simulink model "Auto_microgrid_forecasting"  (R2020a)
settings: Solver=VariableStepAuto  StartTime=0.0  StopTime=40  MaxStep=1e-4  RelTol=1e-3
PreLoadFcn:
  | %load('GC_maxRPP_WS12_GHI790_BL330_nomSOC.mat')
InitFcn:
  | run('FC_microgrid_param.m')
  | tic
  | run('CARTinitFcn.m')
StopFcn:
  | toc
undefined symbols (not defined in the file or in its folder): breakpoints1, breakpoints2, cc_kp, cp_table_data, ctrl, D1, Delta, DiscIntNeverNeededParam, DT, FC_BESS, FC_PV_FirstSolar, find_system, Fnom, forecast, GC_mode, gcbh, GHI_rated, libFC_BESS, libFC_PV, LowerLimit, magnitude, oversize, pll_ki, pll_kp, Pmax_PV, Pmax_WT, sps_rtmsupport, timer, Ts, Ts_APC, Ts_Control, Ts_Power, U_rated, UpperLimit
libraries: powerlib x146, simulink x124, powerlib_extras x120, powerlib_meascontrol x94, eePowerMeasurement x28, pi_ctrl x20, simulink_extras x12, eeGeneralControl x10, sps_avr x7, libFSArray x2, libLgBattery x1, spsDieselMotorModel x1
(part 14 of 16)

== system Auto_microgrid_forecasting/FC_PV_FirstSolar/AllStringInverters/PV_Control/InvControl1/CB_Meas2/Filter1 ==
  In1 : Inport
  Discrete 2nd-Order Filter : powerlib_extras/Discrete  Control Blocks/Discrete  2nd-Order Filter  FilterType=Lowpass  Fo=10  Zeta=0.707  Ts=Ts  Initialize=off  Vac_Init=[0.8 -25 60]  Vdc_Init=-0.4  PlotResponse=off  param1=[1 500 1]
      settings: SourceProductBaseCode=PS
  Discrete 2nd-Order Filter1 : powerlib_extras/Discrete  Control Blocks/Discrete  2nd-Order Filter  FilterType=Lowpass  Fo=10  Zeta=0.707  Ts=Ts  Initialize=off  Vac_Init=[0.8 -25 60]  Vdc_Init=-0.4  PlotResponse=off  param1=[1 500 1]
      settings: SourceProductBaseCode=PS
  Mux : Mux  Inputs=2
  Selector1 : Selector  InputPortWidth=3  IndexOptions=Index vector (dialog)  Indices=1  OutputSizes=1
  Selector2 : Selector  InputPortWidth=3  IndexOptions=Index vector (dialog)  Indices=2  OutputSizes=1
  Out1 : Outport  VectorParamsAs1DForOutWhenUnconnected=off
  wires:
  Mux/1 -> Out1/1  "idq0_line_flt"
  Discrete 2nd-Order Filter1/1 -> Mux/2
  Discrete 2nd-Order Filter/1 -> Mux/1
  Selector1/1 -> Discrete 2nd-Order Filter/1
  Selector2/1 -> Discrete 2nd-Order Filter1/1
  In1/1 -> Selector1/1, Selector2/1

== system Auto_microgrid_forecasting/FC_PV_FirstSolar/AllStringInverters/PV_Control/InvControl1/CB_Meas2/PQ_Calculator ==
  note: Copyright (c) 2016 Massachusetts Institute of Technology
      | Permission is hereby granted, free of charge, to any person obtaining a copy of this software and associated documentation files (the "Software"), to deal
      | in the Software without restriction, including without limitation the rights to use, copy, modify, merge, publish, distribute, sublicense, and/or sell copies of the
      | Software, and to permit persons to whom the Software is furnished to do so, subject to the following conditions:
      |
      | THE SOFTWARE IS PROVIDED "AS IS", WITHOUT WARRANTY OF ANY KIND, EXPRESS OR IMPLIED, INCLUDING BUT NOT LIMITED TO THE
      | WARRANTIES OF MERCHANTABILITY, FITNESS FOR A PARTICULAR PURPOSE AND NONINFRINGEMENT. IN NO EVENT SHALL THE AUTHORS
      | OR COPYRIGHT HOLDERS BE LIABLE FOR ANY CLAIM, DAMAGES OR OTHER LIABILITY, WHETHER IN AN ACTION OF CONTRACT, TORT OR
      | OTHERWISE, ARISING FROM, OUT OF OR IN CONNECTION WITH THE SOFTWARE OR THE USE OR OTHER DEALINGS IN THE SOFTWARE
  Vabc : Inport
  Iabc : Inport  Port=2
  3-phase Instantaneous Active & Reactive Power : powerlib_extras/Measurements/3-phase  Instantaneous  Active & Reactive Power
      settings: SourceProductBaseCode=PS
  Demux : Demux  Outputs=2
  Discrete Mean value2 : powerlib_extras/Discrete Measurements/Discrete  Mean value  Freq=60  Vinit=0  Ts=Ts
      settings: SourceProductBaseCode=PS
  Gain10 : Gain  Gain=2/3
  Scope : Scope  NumInputPorts=4
  P - kW : Outport  VectorParamsAs1DForOutWhenUnconnected=off
  Q - kVAR : Outport  Port=2  VectorParamsAs1DForOutWhenUnconnected=off
  wires:
  Gain10/1 -> Scope/4, Demux/1
  3-phase Instantaneous Active & Reactive Power/1 -> Scope/3, Discrete Mean value2/1
  Discrete Mean value2/1 -> Gain10/1
  Vabc/1 -> Scope/1, 3-phase Instantaneous Active & Reactive Power/1
  Iabc/1 -> Scope/2, 3-phase Instantaneous Active & Reactive Power/2
  Demux/1 -> P - kW/1  "kw"
  Demux/2 -> Q - kVAR/1  "kvar"

== system Auto_microgrid_forecasting/FC_PV_FirstSolar/AllStringInverters/PV_Control/InvControl1/Droop/Droop ==
  dfvpq : Inport
  droop : Inport  Port=2
  Constant4 : Constant  Value=2
  Dead Zone : DeadZone  LowerValue=-1.1  UpperValue=1.1  SaturateOnIntegerOverflow=on
  Demux : Demux
  Demux1 : Demux
  Discrete 1st-Order Filter : powerlib_extras/Discrete  Control Blocks/Discrete 1st-Order Filter  FilterType=Lowpass  Tc=1e-3  Ts=Ts  Initialize=off  Vac_Init=[0.8 -25 60]  Vdc_Init=-0.4  PlotResponse=off  param1=[1 500 0.1]
      settings: SourceProductBaseCode=PS
  Discrete 1st-Order Filter1 : powerlib_extras/Discrete  Control Blocks/Discrete 1st-Order Filter  FilterType=Lowpass  Tc=1e-3  Ts=Ts  Initialize=off  Vac_Init=[0.8 -25 60]  Vdc_Init=-0.4  PlotResponse=off  param1=[1 500 0.1]
      settings: SourceProductBaseCode=PS
  Discrete 2nd-Order Filter : powerlib_extras/Discrete  Control Blocks/Discrete  2nd-Order Filter  FilterType=Lowpass  Fo=100  Zeta=0.707  Ts=Ts  Initialize=off  Vac_Init=[0.8 -25 60]  Vdc_Init=-0.4  PlotResponse=off  param1=[1 500 1]
      settings: SourceProductBaseCode=PS
  Discrete 2nd-Order Filter1 : powerlib_extras/Discrete  Control Blocks/Discrete  2nd-Order Filter  FilterType=Lowpass  Fo=100  Zeta=0.707  Ts=Ts  Initialize=off  Vac_Init=[0.8 -25 60]  Vdc_Init=-0.4  PlotResponse=off  param1=[1 500 1]
      settings: SourceProductBaseCode=PS
  Mux1 : Mux
  Product{,1..4} (5 alike) : Product
  Selector : Selector  InputPortWidth=4  IndexOptions=Index vector (dialog)  Indices=[3 4 1 2]  OutputSizes=1
  Sum : Sum  Inputs=|++
  dFvpq_out : Outport  VectorParamsAs1DForOutWhenUnconnected=off
  wires:
  Product4/1 -> Sum/2
  Sum/1 -> Mux1/4
  Constant4/1 -> Product4/2
  Dead Zone/1 -> Product4/1
  Discrete 2nd-Order Filter/1 -> Product/1
  Discrete 2nd-Order Filter1/1 -> Dead Zone/1, Product2/1
  Demux/3 -> Discrete 2nd-Order Filter/1  "p"
  Discrete 1st-Order Filter/1 -> Product1/1
  Demux/2 -> Discrete 1st-Order Filter1/1  "v"
  Demux/1 -> Discrete 1st-Order Filter/1  "f"
  dfvpq/1 -> Demux/1
  Selector/1 -> dFvpq_out/1
  Discrete 1st-Order Filter1/1 -> Product3/1
  Demux/4 -> Discrete 2nd-Order Filter1/1  "q"
  Product1/1 -> Mux1/1  "p"
  Product3/1 -> Mux1/2  "q"
  Product/1 -> Mux1/3  "F"
  Product2/1 -> Sum/1  "v"
  Mux1/1 -> Selector/1
  Demux1/1 -> Product1/2
  Demux1/4 -> Product2/2
  Demux1/3 -> Product/2
  Demux1/2 -> Product3/2
  droop/1 -> Demux1/1

== system Auto_microgrid_forecasting/FC_PV_FirstSolar/AllStringInverters/PV_Control/InvControl1/Droop/ExtractCoefs ==
  In1 : Inport
  Bus Selector8 : BusSelector  OutputSignals=FP_droop,VQ_droop,FP_droop,VQ_droop
  Mux : Mux
  Out1 : Outport  VectorParamsAs1DForOutWhenUnconnected=off
  wires:
  Bus Selector8/1 -> Mux/1  "<FP_droop>"
  Bus Selector8/4 -> Mux/4  "<VQ_droop>"
  Bus Selector8/2 -> Mux/2  "<VQ_droop>"
  Bus Selector8/3 -> Mux/3  "<FP_droop>"
  Mux/1 -> Out1/1
  In1/1 -> Bus Selector8/1

== system Auto_microgrid_forecasting/FC_PV_FirstSolar/AllStringInverters/PV_Control/InvControl1/PLL/DebounceAlternative ==
  In : Inport
  Rst : Inport  Port=2
  Bias : Bias  Bias=-0.5
  Constant1 : Constant  Value=2/Tdb_on
  Constant2 : Constant  Value=2/Tdb_off
  Data Type Conversion : DataTypeConversion
  Delay : Delay  DelayLength=1  InitialCondition=0
  Discrete-Time Integrator : DiscreteIntegrator  IntegratorMethod=Accumulation: Forward Euler  gainval=Tdb_sample  ExternalReset=level  InitialConditionSource=external  InitialCondition=-0.001  SampleTime=Tdb_sample  OutDataTypeStr=double  LimitOutput=on  UpperSaturationLimit=1.001  LowerSaturationLimit=-0.001  ICPrevOutput=DiscIntNeverNeededParam  ICPrevScaledInput=DiscIntNeverNeededParam
  Logical Operator : Logic  Operator=NXOR  AllPortsSameDT=off  OutDataTypeStr=boolean
  Logical Operator1 : Logic  Operator=OR  AllPortsSameDT=off  OutDataTypeStr=boolean
  Logical Operator2 : Logic  Operator=NOT  AllPortsSameDT=off  OutDataTypeStr=boolean
  Logical Operator3 : Logic  AllPortsSameDT=off  OutDataTypeStr=boolean
  Product : Product
  Relay : Relay  OnSwitchValue=1  OffSwitchValue=0
  Switch : Switch  Threshold=0.5
  Out : Outport  VectorParamsAs1DForOutWhenUnconnected=off
  IntOut : Outport  Port=2  VectorParamsAs1DForOutWhenUnconnected=off
  wires:
  Product/1 -> Discrete-Time Integrator/1
  Relay/1 -> Out/1, Delay/1
  Discrete-Time Integrator/1 -> Relay/1, IntOut/1
  Bias/1 -> Product/1
  Constant1/1 -> Switch/1
  Constant2/1 -> Switch/3
  Delay/1 -> Switch/2, Logical Operator3/2, Logical Operator/2
  Logical Operator/1 -> Logical Operator1/1
  Switch/1 -> Product/2
  In/1 -> Logical Operator/1, Bias/1
  Logical Operator1/1 -> Discrete-Time Integrator/2
  Rst/1 -> Logical Operator2/1, Logical Operator1/2
  Logical Operator3/1 -> Data Type Conversion/1
  Logical Operator2/1 -> Logical Operator3/1
  Data Type Conversion/1 -> Discrete-Time Integrator/3

== system Auto_microgrid_forecasting/FC_PV_FirstSolar/AllStringInverters/PV_Control/InvControl1/PLL/PLL (3ph)1 ==
  abc : Inport  PortDimensions=3
  Discrete : Subsystem  DialogController=POWERSYS.PowerSysDialog  mask(Discrete PID Controller){Kp=ParK(1), Ki=ParK(2), Kd=ParK(3), TcD=TcD, Par_Limits=[Flim(2) Flim(1)]*2*pi, Init=2*pi*Par_Init(2), Ts=Ts}
      mask prompts: Kp "Proportional gain (Kp):"; Ki "Integral gain (Ki):"; Kd "Derivative gain (Kd):"; TcD "Time constant for derivative filter (s):"; Par_Limits "Output limits: [ Upper   Lower ]"; Init "Output initial value:"; Ts "Sample time:"
      mask help: This block implements a discrete PID controller.
      mask Display: disp('PID');
  Discrete 2nd-Order Filter : powerlib_extras/Discrete  Control Blocks/Discrete  2nd-Order Filter  FilterType=Lowpass  Fo=10  Zeta=0.707  Ts=Ts  Initialize=off  Vac_Init=[0.8 -25 60]  Vdc_Init=-0.4  PlotResponse=off  param1=[1 500 1]
      settings: SourceProductBaseCode=PS
  Gain10 : Gain  Gain=1/2/pi  SaturateOnIntegerOverflow=on  OutDataTypeStr=Inherit: Same as input  ParamDataTypeStr=Inherit: Same as input
  Mux3 : Mux  Inputs=2
  Scope : Scope  NumInputPorts=4
  Selector : Selector  InputPortWidth=3  IndexOptions=Index vector (dialog)  Indices=2  OutputSizes=1
  Trigonometric Function2 : Trigonometry
  Trigonometric Function3 : Trigonometry  Operator=cos
  Unit Delay : UnitDelay  SampleTime=Ts  HasFrameUpgradeWarning=on
  VCO : Subsystem
  abc_to_dq0 Transformation : powerlib_extras/Measurements/abc_to_dq0 Transformation
      settings: SourceProductBaseCode=PS
  Freq : Outport  VectorParamsAs1DForOutWhenUnconnected=off
  wt : Outport  Port=2  VectorParamsAs1DForOutWhenUnconnected=off
  dq0 : Outport  Port=3  VectorParamsAs1DForOutWhenUnconnected=off
  wires:
  Trigonometric Function3/1 -> Mux3/2
  Trigonometric Function2/1 -> Mux3/1
  Mux3/1 -> abc_to_dq0 Transformation/2  "ejwt"
  abc_to_dq0 Transformation/1 -> dq0/1, Selector/1
  abc/1 -> Scope/4, abc_to_dq0 Transformation/1
  Discrete 2nd-Order Filter/1 -> Unit Delay/1
  Selector/1 -> Scope/1, Discrete/1(Err)  "Vq"
  Gain10/1 -> Discrete 2nd-Order Filter/1
  Unit Delay/1 -> Freq/1
  Discrete/1(Out) -> Scope/2, VCO/1(w), Gain10/1  "W"
  VCO/1(theta) -> Trigonometric Function2/1, Trigonometric Function3/1, wt/1, Scope/3  "wt"

== system Auto_microgrid_forecasting/FC_PV_FirstSolar/AllStringInverters/PV_Control/InvControl1/PLL/VCO ==
  w : Inport
  rst : Inport  Port=2
  init : Inport  Port=3
  Compare To Constant : simulink/Logic and Bit Operations/Compare To Constant  relop=>=  const=pi  OutDataTypeStr=uint8
  Data Type Conversion : DataTypeConversion
  Gain : Gain  Gain=2*pi  OutDataTypeStr=double
  Gain2 : Gain  Gain=Ts  SaturateOnIntegerOverflow=on  OutDataTypeStr=Inherit: Same as input  ParamDataTypeStr=Inherit: Same as input
  Sum : Sum  Inputs=-++
  Switch : Switch  Threshold=0.5
  Unit Delay1 : UnitDelay  SampleTime=-1  HasFrameUpgradeWarning=on
  theta : Outport  VectorParamsAs1DForOutWhenUnconnected=off
  wires:
  Data Type Conversion/1 -> Gain/1
  init/1 -> Switch/1
  rst/1 -> Switch/2
  Switch/1 -> Unit Delay1/1
  Sum/1 -> Switch/3
  Gain2/1 -> Sum/2
  Unit Delay1/1 -> Compare To Constant/1, theta/1, Sum/3  "wt"
  Compare To Constant/1 -> Data Type Conversion/1
  Gain/1 -> Sum/1
  w/1 -> Gain2/1

== system Auto_microgrid_forecasting/FC_PV_FirstSolar/AllStringInverters/PV_Control/InvControl1/Ref_Limiting/RefLimiting ==
  fvpq_in : Inport
  p_max : Inport  Port=2
  p_min : Inport  Port=3
  Complex to Magnitude-Angle : ComplexToMagnitudeAngle
  Complex to Real-Imag : ComplexToRealImag
  Demux : Demux
  Magnitude-Angle to Complex : MagnitudeAngleToComplex
  Mux2 : Mux
  Real-Imag to Complex : RealImagToComplex
  Saturation : Saturate  UpperLimit=1.1  LowerLimit=0.9
  Saturation Dynamic : simulink/Discontinuities/Saturation Dynamic  OutMin=[]  OutMax=[]  OutDataTypeStr=Inherit: Same as second input  OutDataType=fixdt(1, 16)  OutScaling=2^-10  DoSatur=off
  Saturation1 : Saturate  UpperLimit=1.5  LowerLimit=00
  Saturation2 : Saturate  UpperLimit=1  LowerLimit=0
  fvpq_out : Outport  VectorParamsAs1DForOutWhenUnconnected=off
  wires:
  p_min/1 -> Saturation Dynamic/3
  Saturation1/1 -> Mux2/2
  Magnitude-Angle to Complex/1 -> Complex to Real-Imag/1
  Mux2/1 -> fvpq_out/1  "fvpq"
  Demux/3 -> Saturation Dynamic/2
  Saturation Dynamic/1 -> Real-Imag to Complex/1
  Complex to Magnitude-Angle/1 -> Saturation2/1
  Complex to Real-Imag/2 -> Mux2/4
  Complex to Real-Imag/1 -> Mux2/3
  Real-Imag to Complex/1 -> Complex to Magnitude-Angle/1
  Demux/2 -> Saturation1/1
  Demux/1 -> Saturation/1
  fvpq_in/1 -> Demux/1
  Saturation2/1 -> Magnitude-Angle to Complex/1
  Saturation/1 -> Mux2/1
  p_max/1 -> Saturation Dynamic/1
  Complex to Magnitude-Angle/2 -> Magnitude-Angle to Complex/2
  Demux/4 -> Real-Imag to Complex/2

== system Auto_microgrid_forecasting/FC_PV_FirstSolar/AllStringInverters/PV_Control/InvControl2/40_V_Control/Subsystem ==
  in : Inport
  rst : Inport  Port=2
  init : Inport  Port=3
  rate : Inport  Port=4
  Gain : Gain  Gain=[Ts Ts]
  Gain1 : Gain  Gain=-1
  Saturation Dynamic : simulink/Discontinuities/Saturation Dynamic  OutMin=[]  OutMax=[]  OutDataTypeStr=Inherit: Same as second input  OutDataType=fixdt(1, 16)  OutScaling=2^-10  DoSatur=off
  Sum : Sum  Inputs=|++
  Sum1 : Sum  Inputs=-+|
  Switch : Switch  Criteria=u2 > Threshold
  Unit Delay : UnitDelay  SampleTime=-1  HasFrameUpgradeWarning=on
  out : Outport  VectorParamsAs1DForOutWhenUnconnected=off
  wires:
  Switch/1 -> Unit Delay/1
  Sum/1 -> Switch/3
  Saturation Dynamic/1 -> Sum/1
  in/1 -> Sum1/2
  Sum1/1 -> Saturation Dynamic/2
  rst/1 -> Switch/2
  init/1 -> Switch/1
  Unit Delay/1 -> Sum/2, Sum1/1, out/1
  rate/1 -> Gain/1
  Gain/1 -> Saturation Dynamic/1, Gain1/1
  Gain1/1 -> Saturation Dynamic/3

== system Auto_microgrid_forecasting/FC_PV_FirstSolar/AllStringInverters/PV_Control/InvControl2/50_I_Control/Filter ==
  In1 : Inport
  Discrete 2nd-Order Filter : powerlib_extras/Discrete  Control Blocks/Discrete  2nd-Order Filter  FilterType=Lowpass  Fo=300  Zeta=0.707  Ts=Ts  Initialize=off  Vac_Init=[0.8 -25 60]  Vdc_Init=-0.4  PlotResponse=off  param1=[1 500 1]
      settings: SourceProductBaseCode=PS
  Discrete 2nd-Order Filter1 : powerlib_extras/Discrete  Control Blocks/Discrete  2nd-Order Filter  FilterType=Lowpass  Fo=300  Zeta=0.707  Ts=Ts  Initialize=off  Vac_Init=[0.8 -25 60]  Vdc_Init=-0.4  PlotResponse=off  param1=[1 500 1]
      settings: SourceProductBaseCode=PS
  Mux : Mux  Inputs=2
  Selector1 : Selector  InputPortWidth=2  IndexOptions=Index vector (dialog)  Indices=1  OutputSizes=1
  Selector2 : Selector  InputPortWidth=2  IndexOptions=Index vector (dialog)  Indices=2  OutputSizes=1
  Out1 : Outport  VectorParamsAs1DForOutWhenUnconnected=off
  wires:
  In1/1 -> Selector2/1, Selector1/1
  Selector2/1 -> Discrete 2nd-Order Filter1/1
  Selector1/1 -> Discrete 2nd-Order Filter/1
  Discrete 2nd-Order Filter/1 -> Mux/1
  Discrete 2nd-Order Filter1/1 -> Mux/2
  Mux/1 -> Out1/1  "vdq0_line_flt"

== system Auto_microgrid_forecasting/FC_PV_FirstSolar/AllStringInverters/PV_Control/InvControl2/50_I_Control/Filter1 ==
  In1 : Inport
  Discrete 2nd-Order Filter : powerlib_extras/Discrete  Control Blocks/Discrete  2nd-Order Filter  FilterType=Lowpass  Fo=40  Zeta=1  Ts=Ts  Initialize=off  Vac_Init=[0.8 -25 60]  Vdc_Init=-0.4  PlotResponse=off  param1=[1 500 1]
      settings: SourceProductBaseCode=PS
  Discrete 2nd-Order Filter1 : powerlib_extras/Discrete  Control Blocks/Discrete  2nd-Order Filter  FilterType=Lowpass  Fo=40  Zeta=1  Ts=Ts  Initialize=off  Vac_Init=[0.8 -25 60]  Vdc_Init=-0.4  PlotResponse=off  param1=[1 500 1]
      settings: SourceProductBaseCode=PS
  Mux : Mux  Inputs=2
  Selector1 : Selector  InputPortWidth=2  IndexOptions=Index vector (dialog)  Indices=1  OutputSizes=1
  Selector2 : Selector  InputPortWidth=2  IndexOptions=Index vector (dialog)  Indices=2  OutputSizes=1
  Out1 : Outport  VectorParamsAs1DForOutWhenUnconnected=off
  wires:
  Mux/1 -> Out1/1  "vdq0_line_flt"
  Discrete 2nd-Order Filter1/1 -> Mux/2
  Discrete 2nd-Order Filter/1 -> Mux/1
  Selector1/1 -> Discrete 2nd-Order Filter/1
  Selector2/1 -> Discrete 2nd-Order Filter1/1
  In1/1 -> Selector1/1, Selector2/1

== system Auto_microgrid_forecasting/FC_PV_FirstSolar/AllStringInverters/PV_Control/InvControl2/50_I_Control/Subsystem ==
  in : Inport
  rst : Inport  Port=2
  init : Inport  Port=3
  rate : Inport  Port=4
  Gain : Gain  Gain=[Ts Ts]
  Gain1 : Gain  Gain=-1
  Saturation Dynamic : simulink/Discontinuities/Saturation Dynamic  OutMin=[]  OutMax=[]  OutDataTypeStr=Inherit: Same as second input  OutDataType=fixdt(1, 16)  OutScaling=2^-10  DoSatur=off
  Sum : Sum  Inputs=|++
  Sum1 : Sum  Inputs=-+|
  Switch : Switch  Criteria=u2 > Threshold
  Unit Delay : UnitDelay  SampleTime=-1  HasFrameUpgradeWarning=on
  out : Outport  VectorParamsAs1DForOutWhenUnconnected=off
  wires:
  Switch/1 -> Unit Delay/1
  Sum/1 -> Switch/3
  Saturation Dynamic/1 -> Sum/1
  in/1 -> Sum1/2
  Sum1/1 -> Saturation Dynamic/2
  rst/1 -> Switch/2
  init/1 -> Switch/1
  Unit Delay/1 -> Sum/2, Sum1/1, out/1
  rate/1 -> Gain/1
  Gain/1 -> Saturation Dynamic/1, Gain1/1
  Gain1/1 -> Saturation Dynamic/3

== system Auto_microgrid_forecasting/FC_PV_FirstSolar/AllStringInverters/PV_Control/InvControl2/CB_Meas2/Filter ==
  In1 : Inport
  Discrete 2nd-Order Filter : powerlib_extras/Discrete  Control Blocks/Discrete  2nd-Order Filter  FilterType=Lowpass  Fo=10  Zeta=0.707  Ts=Ts  Initialize=off  Vac_Init=[0.8 -25 60]  Vdc_Init=-0.4  PlotResponse=off  param1=[1 500 1]
      settings: SourceProductBaseCode=PS
  Discrete 2nd-Order Filter1 : powerlib_extras/Discrete  Control Blocks/Discrete  2nd-Order Filter  FilterType=Lowpass  Fo=10  Zeta=0.707  Ts=Ts  Initialize=off  Vac_Init=[0.8 -25 60]  Vdc_Init=-0.4  PlotResponse=off  param1=[1 500 1]
      settings: SourceProductBaseCode=PS
  Mux : Mux  Inputs=2
  Selector1 : Selector  InputPortWidth=3  IndexOptions=Index vector (dialog)  Indices=1  OutputSizes=1
  Selector2 : Selector  InputPortWidth=3  IndexOptions=Index vector (dialog)  Indices=2  OutputSizes=1
  Out1 : Outport  VectorParamsAs1DForOutWhenUnconnected=off
  wires:
  In1/1 -> Selector2/1, Selector1/1
  Selector2/1 -> Discrete 2nd-Order Filter1/1
  Selector1/1 -> Discrete 2nd-Order Filter/1
  Discrete 2nd-Order Filter/1 -> Mux/1
  Discrete 2nd-Order Filter1/1 -> Mux/2
  Mux/1 -> Out1/1  "vdq0_line_flt"

== system Auto_microgrid_forecasting/FC_PV_FirstSolar/AllStringInverters/PV_Control/InvControl2/CB_Meas2/Filter1 ==
  In1 : Inport
  Discrete 2nd-Order Filter : powerlib_extras/Discrete  Control Blocks/Discrete  2nd-Order Filter  FilterType=Lowpass  Fo=10  Zeta=0.707  Ts=Ts  Initialize=off  Vac_Init=[0.8 -25 60]  Vdc_Init=-0.4  PlotResponse=off  param1=[1 500 1]
      settings: SourceProductBaseCode=PS
  Discrete 2nd-Order Filter1 : powerlib_extras/Discrete  Control Blocks/Discrete  2nd-Order Filter  FilterType=Lowpass  Fo=10  Zeta=0.707  Ts=Ts  Initialize=off  Vac_Init=[0.8 -25 60]  Vdc_Init=-0.4  PlotResponse=off  param1=[1 500 1]
      settings: SourceProductBaseCode=PS
  Mux : Mux  Inputs=2
  Selector1 : Selector  InputPortWidth=3  IndexOptions=Index vector (dialog)  Indices=1  OutputSizes=1
  Selector2 : Selector  InputPortWidth=3  IndexOptions=Index vector (dialog)  Indices=2  OutputSizes=1
  Out1 : Outport  VectorParamsAs1DForOutWhenUnconnected=off
  wires:
  In1/1 -> Selector2/1, Selector1/1
  Selector2/1 -> Discrete 2nd-Order Filter1/1
  Selector1/1 -> Discrete 2nd-Order Filter/1
  Discrete 2nd-Order Filter/1 -> Mux/1
  Discrete 2nd-Order Filter1/1 -> Mux/2
  Mux/1 -> Out1/1  "idq0_line_flt"

== system Auto_microgrid_forecasting/FC_PV_FirstSolar/AllStringInverters/PV_Control/InvControl2/CB_Meas2/PQ_Calculator ==
  note: Copyright (c) 2016 Massachusetts Institute of Technology
      | Permission is hereby granted, free of charge, to any person obtaining a copy of this software and associated documentation files (the "Software"), to deal
      | in the Software without restriction, including without limitation the rights to use, copy, modify, merge, publish, distribute, sublicense, and/or sell copies of the
      | Software, and to permit persons to whom the Software is furnished to do so, subject to the following conditions:
      |
      | THE SOFTWARE IS PROVIDED "AS IS", WITHOUT WARRANTY OF ANY KIND, EXPRESS OR IMPLIED, INCLUDING BUT NOT LIMITED TO THE
      | WARRANTIES OF MERCHANTABILITY, FITNESS FOR A PARTICULAR PURPOSE AND NONINFRINGEMENT. IN NO EVENT SHALL THE AUTHORS
      | OR COPYRIGHT HOLDERS BE LIABLE FOR ANY CLAIM, DAMAGES OR OTHER LIABILITY, WHETHER IN AN ACTION OF CONTRACT, TORT OR
      | OTHERWISE, ARISING FROM, OUT OF OR IN CONNECTION WITH THE SOFTWARE OR THE USE OR OTHER DEALINGS IN THE SOFTWARE
  Vabc : Inport
  Iabc : Inport  Port=2
  3-phase Instantaneous Active & Reactive Power : powerlib_extras/Measurements/3-phase  Instantaneous  Active & Reactive Power
      settings: SourceProductBaseCode=PS
  Demux : Demux  Outputs=2
  Discrete Mean value2 : powerlib_extras/Discrete Measurements/Discrete  Mean value  Freq=60  Vinit=0  Ts=Ts
      settings: SourceProductBaseCode=PS
  Gain10 : Gain  Gain=2/3
  Scope : Scope  NumInputPorts=4
  P - kW : Outport  VectorParamsAs1DForOutWhenUnconnected=off
  Q - kVAR : Outport  Port=2  VectorParamsAs1DForOutWhenUnconnected=off
  wires:
  Demux/2 -> Q - kVAR/1  "kvar"
  Demux/1 -> P - kW/1  "kw"
  Iabc/1 -> 3-phase Instantaneous Active & Reactive Power/2, Scope/2
  Vabc/1 -> 3-phase Instantaneous Active & Reactive Power/1, Scope/1
  Discrete Mean value2/1 -> Gain10/1
  3-phase Instantaneous Active & Reactive Power/1 -> Discrete Mean value2/1, Scope/3
  Gain10/1 -> Demux/1, Scope/4

== system Auto_microgrid_forecasting/FC_PV_FirstSolar/AllStringInverters/PV_Control/InvControl2/Droop/Droop ==
  dfvpq : Inport
  droop : Inport  Port=2
  Constant4 : Constant  Value=2
  Dead Zone : DeadZone  LowerValue=-1.1  UpperValue=1.1  SaturateOnIntegerOverflow=on
  Demux : Demux
  Demux1 : Demux
  Discrete 1st-Order Filter : powerlib_extras/Discrete  Control Blocks/Discrete 1st-Order Filter  FilterType=Lowpass  Tc=1e-3  Ts=Ts  Initialize=off  Vac_Init=[0.8 -25 60]  Vdc_Init=-0.4  PlotResponse=off  param1=[1 500 0.1]
      settings: SourceProductBaseCode=PS
  Discrete 1st-Order Filter1 : powerlib_extras/Discrete  Control Blocks/Discrete 1st-Order Filter  FilterType=Lowpass  Tc=1e-3  Ts=Ts  Initialize=off  Vac_Init=[0.8 -25 60]  Vdc_Init=-0.4  PlotResponse=off  param1=[1 500 0.1]
      settings: SourceProductBaseCode=PS
  Discrete 2nd-Order Filter : powerlib_extras/Discrete  Control Blocks/Discrete  2nd-Order Filter  FilterType=Lowpass  Fo=100  Zeta=0.707  Ts=Ts  Initialize=off  Vac_Init=[0.8 -25 60]  Vdc_Init=-0.4  PlotResponse=off  param1=[1 500 1]
      settings: SourceProductBaseCode=PS
  Discrete 2nd-Order Filter1 : powerlib_extras/Discrete  Control Blocks/Discrete  2nd-Order Filter  FilterType=Lowpass  Fo=100  Zeta=0.707  Ts=Ts  Initialize=off  Vac_Init=[0.8 -25 60]  Vdc_Init=-0.4  PlotResponse=off  param1=[1 500 1]
      settings: SourceProductBaseCode=PS
  Mux1 : Mux
  Product{,1..4} (5 alike) : Product
  Selector : Selector  InputPortWidth=4  IndexOptions=Index vector (dialog)  Indices=[3 4 1 2]  OutputSizes=1
  Sum : Sum  Inputs=|++
  dFvpq_out : Outport  VectorParamsAs1DForOutWhenUnconnected=off
  wires:
  droop/1 -> Demux1/1
  Demux1/2 -> Product3/2
  Demux1/3 -> Product/2
  Demux1/4 -> Product2/2
  Demux1/1 -> Product1/2
  Mux1/1 -> Selector/1
  Product2/1 -> Sum/1  "v"
  Product/1 -> Mux1/3  "F"
  Product3/1 -> Mux1/2  "q"
  Product1/1 -> Mux1/1  "p"
  Demux/4 -> Discrete 2nd-Order Filter1/1  "q"
  Discrete 1st-Order Filter1/1 -> Product3/1
  Selector/1 -> dFvpq_out/1
  dfvpq/1 -> Demux/1
  Demux/1 -> Discrete 1st-Order Filter/1  "f"
  Demux/2 -> Discrete 1st-Order Filter1/1  "v"
  Discrete 1st-Order Filter/1 -> Product1/1
  Demux/3 -> Discrete 2nd-Order Filter/1  "p"
  Discrete 2nd-Order Filter1/1 -> Product2/1, Dead Zone/1
  Discrete 2nd-Order Filter/1 -> Product/1
  Dead Zone/1 -> Product4/1
  Constant4/1 -> Product4/2
  Sum/1 -> Mux1/4
  Product4/1 -> Sum/2

== system Auto_microgrid_forecasting/FC_PV_FirstSolar/AllStringInverters/PV_Control/InvControl2/Droop/ExtractCoefs ==
  In1 : Inport
  Bus Selector8 : BusSelector  OutputSignals=FP_droop,VQ_droop,FP_droop,VQ_droop
  Mux : Mux
  Out1 : Outport  VectorParamsAs1DForOutWhenUnconnected=off
  wires:
  In1/1 -> Bus Selector8/1
  Mux/1 -> Out1/1
  Bus Selector8/3 -> Mux/3  "<FP_droop>"
  Bus Selector8/2 -> Mux/2  "<VQ_droop>"
  Bus Selector8/4 -> Mux/4  "<VQ_droop>"
  Bus Selector8/1 -> Mux/1  "<FP_droop>"

== system Auto_microgrid_forecasting/FC_PV_FirstSolar/AllStringInverters/PV_Control/InvControl2/PLL/DebounceAlternative ==
  In : Inport
  Rst : Inport  Port=2
  Bias : Bias  Bias=-0.5
  Constant1 : Constant  Value=2/Tdb_on
  Constant2 : Constant  Value=2/Tdb_off
  Data Type Conversion : DataTypeConversion
  Delay : Delay  DelayLength=1  InitialCondition=0
  Discrete-Time Integrator : DiscreteIntegrator  IntegratorMethod=Accumulation: Forward Euler  gainval=Tdb_sample  ExternalReset=level  InitialConditionSource=external  InitialCondition=-0.001  SampleTime=Tdb_sample  OutDataTypeStr=double  LimitOutput=on  UpperSaturationLimit=1.001  LowerSaturationLimit=-0.001  ICPrevOutput=DiscIntNeverNeededParam  ICPrevScaledInput=DiscIntNeverNeededParam
  Logical Operator : Logic  Operator=NXOR  AllPortsSameDT=off  OutDataTypeStr=boolean
  Logical Operator1 : Logic  Operator=OR  AllPortsSameDT=off  OutDataTypeStr=boolean
  Logical Operator2 : Logic  Operator=NOT  AllPortsSameDT=off  OutDataTypeStr=boolean
  Logical Operator3 : Logic  AllPortsSameDT=off  OutDataTypeStr=boolean
  Product : Product
  Relay : Relay  OnSwitchValue=1  OffSwitchValue=0
  Switch : Switch  Threshold=0.5
  Out : Outport  VectorParamsAs1DForOutWhenUnconnected=off
  IntOut : Outport  Port=2  VectorParamsAs1DForOutWhenUnconnected=off
  wires:
  Data Type Conversion/1 -> Discrete-Time Integrator/3
  Logical Operator2/1 -> Logical Operator3/1
  Logical Operator3/1 -> Data Type Conversion/1
  Rst/1 -> Logical Operator1/2, Logical Operator2/1
  Logical Operator1/1 -> Discrete-Time Integrator/2
  In/1 -> Bias/1, Logical Operator/1
  Switch/1 -> Product/2
  Logical Operator/1 -> Logical Operator1/1
  Delay/1 -> Logical Operator/2, Logical Operator3/2, Switch/2
  Constant2/1 -> Switch/3
  Constant1/1 -> Switch/1
  Bias/1 -> Product/1
  Discrete-Time Integrator/1 -> IntOut/1, Relay/1
  Relay/1 -> Delay/1, Out/1
  Product/1 -> Discrete-Time Integrator/1

== system Auto_microgrid_forecasting/FC_PV_FirstSolar/AllStringInverters/PV_Control/InvControl2/PLL/PLL (3ph)1 ==
  abc : Inport  PortDimensions=3
  Discrete : Subsystem  DialogController=POWERSYS.PowerSysDialog  mask(Discrete PID Controller){Kp=ParK(1), Ki=ParK(2), Kd=ParK(3), TcD=TcD, Par_Limits=[Flim(2) Flim(1)]*2*pi, Init=2*pi*Par_Init(2), Ts=Ts}
      mask prompts: Kp "Proportional gain (Kp):"; Ki "Integral gain (Ki):"; Kd "Derivative gain (Kd):"; TcD "Time constant for derivative filter (s):"; Par_Limits "Output limits: [ Upper   Lower ]"; Init "Output initial value:"; Ts "Sample time:"
      mask help: This block implements a discrete PID controller.
      mask Display: disp('PID');
  Discrete 2nd-Order Filter : powerlib_extras/Discrete  Control Blocks/Discrete  2nd-Order Filter  FilterType=Lowpass  Fo=10  Zeta=0.707  Ts=Ts  Initialize=off  Vac_Init=[0.8 -25 60]  Vdc_Init=-0.4  PlotResponse=off  param1=[1 500 1]
      settings: SourceProductBaseCode=PS
  Gain10 : Gain  Gain=1/2/pi  SaturateOnIntegerOverflow=on  OutDataTypeStr=Inherit: Same as input  ParamDataTypeStr=Inherit: Same as input
  Mux3 : Mux  Inputs=2
  Scope : Scope  NumInputPorts=4
  Selector : Selector  InputPortWidth=3  IndexOptions=Index vector (dialog)  Indices=2  OutputSizes=1
  Trigonometric Function2 : Trigonometry
  Trigonometric Function3 : Trigonometry  Operator=cos
  Unit Delay : UnitDelay  SampleTime=Ts  HasFrameUpgradeWarning=on
  VCO : Subsystem
  abc_to_dq0 Transformation : powerlib_extras/Measurements/abc_to_dq0 Transformation
      settings: SourceProductBaseCode=PS
  Freq : Outport  VectorParamsAs1DForOutWhenUnconnected=off
  wt : Outport  Port=2  VectorParamsAs1DForOutWhenUnconnected=off
  dq0 : Outport  Port=3  VectorParamsAs1DForOutWhenUnconnected=off
  wires:
  VCO/1(theta) -> Scope/3, wt/1, Trigonometric Function3/1, Trigonometric Function2/1  "wt"
  Discrete/1(Out) -> Gain10/1, VCO/1(w), Scope/2  "W"
  Unit Delay/1 -> Freq/1
  Gain10/1 -> Discrete 2nd-Order Filter/1
  Selector/1 -> Discrete/1(Err), Scope/1  "Vq"
  Discrete 2nd-Order Filter/1 -> Unit Delay/1
  abc/1 -> abc_to_dq0 Transformation/1, Scope/4
  abc_to_dq0 Transformation/1 -> Selector/1, dq0/1
  Mux3/1 -> abc_to_dq0 Transformation/2  "ejwt"
  Trigonometric Function2/1 -> Mux3/1
  Trigonometric Function3/1 -> Mux3/2

== system Auto_microgrid_forecasting/FC_PV_FirstSolar/AllStringInverters/PV_Control/InvControl2/PLL/VCO ==
  w : Inport
  rst : Inport  Port=2
  init : Inport  Port=3
  Compare To Constant : simulink/Logic and Bit Operations/Compare To Constant  relop=>=  const=pi  OutDataTypeStr=uint8
  Data Type Conversion : DataTypeConversion
  Gain : Gain  Gain=2*pi  OutDataTypeStr=double
  Gain2 : Gain  Gain=Ts  SaturateOnIntegerOverflow=on  OutDataTypeStr=Inherit: Same as input  ParamDataTypeStr=Inherit: Same as input
  Sum : Sum  Inputs=-++
  Switch : Switch  Threshold=0.5
  Unit Delay1 : UnitDelay  SampleTime=-1  HasFrameUpgradeWarning=on
  theta : Outport  VectorParamsAs1DForOutWhenUnconnected=off
  wires:
  w/1 -> Gain2/1
  Gain/1 -> Sum/1
  Compare To Constant/1 -> Data Type Conversion/1
  Unit Delay1/1 -> Sum/3, theta/1, Compare To Constant/1  "wt"
  Gain2/1 -> Sum/2
  Sum/1 -> Switch/3
  Switch/1 -> Unit Delay1/1
  rst/1 -> Switch/2
  init/1 -> Switch/1
  Data Type Conversion/1 -> Gain/1

== system Auto_microgrid_forecasting/FC_PV_FirstSolar/AllStringInverters/PV_Control/InvControl2/Ref_Limiting/RefLimiting ==
  fvpq_in : Inport
  p_max : Inport  Port=2
  p_min : Inport  Port=3
  Complex to Magnitude-Angle : ComplexToMagnitudeAngle
  Complex to Real-Imag : ComplexToRealImag
  Demux : Demux
  Magnitude-Angle to Complex : MagnitudeAngleToComplex
  Mux2 : Mux
  Real-Imag to Complex : RealImagToComplex
  Saturation : Saturate  UpperLimit=1.1  LowerLimit=0.9
  Saturation Dynamic : simulink/Discontinuities/Saturation Dynamic  OutMin=[]  OutMax=[]  OutDataTypeStr=Inherit: Same as second input  OutDataType=fixdt(1, 16)  OutScaling=2^-10  DoSatur=off
  Saturation1 : Saturate  UpperLimit=1.5  LowerLimit=00
  Saturation2 : Saturate  UpperLimit=1  LowerLimit=0
  fvpq_out : Outport  VectorParamsAs1DForOutWhenUnconnected=off
  wires:
  Demux/4 -> Real-Imag to Complex/2
  Complex to Magnitude-Angle/2 -> Magnitude-Angle to Complex/2
  p_max/1 -> Saturation Dynamic/1
  Saturation/1 -> Mux2/1
  Saturation2/1 -> Magnitude-Angle to Complex/1
  fvpq_in/1 -> Demux/1
  Demux/1 -> Saturation/1
  Demux/2 -> Saturation1/1
  Real-Imag to Complex/1 -> Complex to Magnitude-Angle/1
  Complex to Real-Imag/1 -> Mux2/3
  Complex to Real-Imag/2 -> Mux2/4
  Complex to Magnitude-Angle/1 -> Saturation2/1
  Saturation Dynamic/1 -> Real-Imag to Complex/1
  Demux/3 -> Saturation Dynamic/2
  Mux2/1 -> fvpq_out/1  "fvpq"
  Magnitude-Angle to Complex/1 -> Complex to Real-Imag/1
  Saturation1/1 -> Mux2/2
  p_min/1 -> Saturation Dynamic/3

== system Auto_microgrid_forecasting/MODEL STABILIZER/AllStringInverters/Stab_control/InvControl/40_V_Control/Subsystem ==
  in : Inport
  rst : Inport  Port=2
  init : Inport  Port=3
  rate : Inport  Port=4
  Gain : Gain  Gain=[Ts Ts]
  Gain1 : Gain  Gain=-1
  Saturation Dynamic : simulink/Discontinuities/Saturation Dynamic  OutMin=[]  OutMax=[]  OutDataTypeStr=Inherit: Same as second input  OutDataType=fixdt(1, 16)  OutScaling=2^-10  DoSatur=off
  Sum : Sum  Inputs=|++
  Sum1 : Sum  Inputs=-+|
  Switch : Switch  Criteria=u2 > Threshold
  Unit Delay : UnitDelay  SampleTime=-1  HasFrameUpgradeWarning=on
  out : Outport  VectorParamsAs1DForOutWhenUnconnected=off
  wires:
  Switch/1 -> Unit Delay/1
  Sum/1 -> Switch/3
  Saturation Dynamic/1 -> Sum/1
  in/1 -> Sum1/2
  Sum1/1 -> Saturation Dynamic/2
  rst/1 -> Switch/2
  init/1 -> Switch/1
  Unit Delay/1 -> Sum/2, Sum1/1, out/1
  rate/1 -> Gain/1
  Gain/1 -> Saturation Dynamic/1, Gain1/1
  Gain1/1 -> Saturation Dynamic/3

== system Auto_microgrid_forecasting/MODEL STABILIZER/AllStringInverters/Stab_control/InvControl/50_I_Control/Filter ==
  In1 : Inport
  Discrete 2nd-Order Filter : powerlib_extras/Discrete  Control Blocks/Discrete  2nd-Order Filter  FilterType=Lowpass  Fo=1000  Zeta=0.707  Ts=Ts  Initialize=off  Vac_Init=[0.8 -25 60]  Vdc_Init=-0.4  PlotResponse=off  param1=[1 500 1]
      settings: SourceProductBaseCode=PS
  Discrete 2nd-Order Filter1 : powerlib_extras/Discrete  Control Blocks/Discrete  2nd-Order Filter  FilterType=Lowpass  Fo=1000  Zeta=0.707  Ts=Ts  Initialize=off  Vac_Init=[0.8 -25 60]  Vdc_Init=-0.4  PlotResponse=off  param1=[1 500 1]
      settings: SourceProductBaseCode=PS
  Mux : Mux  Inputs=2
  Selector1 : Selector  InputPortWidth=2  IndexOptions=Index vector (dialog)  Indices=1  OutputSizes=1
  Selector2 : Selector  InputPortWidth=2  IndexOptions=Index vector (dialog)  Indices=2  OutputSizes=1
  Out1 : Outport  VectorParamsAs1DForOutWhenUnconnected=off
  wires:
  In1/1 -> Selector2/1, Selector1/1
  Selector2/1 -> Discrete 2nd-Order Filter1/1
  Selector1/1 -> Discrete 2nd-Order Filter/1
  Discrete 2nd-Order Filter/1 -> Mux/1
  Discrete 2nd-Order Filter1/1 -> Mux/2
  Mux/1 -> Out1/1  "vdq0_line_flt"

== system Auto_microgrid_forecasting/MODEL STABILIZER/AllStringInverters/Stab_control/InvControl/50_I_Control/Filter1 ==
  In1 : Inport
  Discrete 2nd-Order Filter : powerlib_extras/Discrete  Control Blocks/Discrete  2nd-Order Filter  FilterType=Lowpass  Fo=500  Zeta=1  Ts=Ts  Initialize=off  Vac_Init=[0.8 -25 60]  Vdc_Init=-0.4  PlotResponse=off  param1=[1 500 1]
      settings: SourceProductBaseCode=PS
  Discrete 2nd-Order Filter1 : powerlib_extras/Discrete  Control Blocks/Discrete  2nd-Order Filter  FilterType=Lowpass  Fo=500  Zeta=1  Ts=Ts  Initialize=off  Vac_Init=[0.8 -25 60]  Vdc_Init=-0.4  PlotResponse=off  param1=[1 500 1]
      settings: SourceProductBaseCode=PS
  Mux : Mux  Inputs=2
  Selector1 : Selector  InputPortWidth=2  IndexOptions=Index vector (dialog)  Indices=1  OutputSizes=1
  Selector2 : Selector  InputPortWidth=2  IndexOptions=Index vector (dialog)  Indices=2  OutputSizes=1
  Out1 : Outport  VectorParamsAs1DForOutWhenUnconnected=off
  wires:
  Mux/1 -> Out1/1  "vdq0_line_flt"
  Discrete 2nd-Order Filter1/1 -> Mux/2
  Discrete 2nd-Order Filter/1 -> Mux/1
  Selector1/1 -> Discrete 2nd-Order Filter/1
  Selector2/1 -> Discrete 2nd-Order Filter1/1
  In1/1 -> Selector1/1, Selector2/1

== system Auto_microgrid_forecasting/MODEL STABILIZER/AllStringInverters/Stab_control/InvControl/50_I_Control/Subsystem ==
  in : Inport
  rst : Inport  Port=2
  init : Inport  Port=3
  rate : Inport  Port=4
  Gain : Gain  Gain=[Ts Ts]
  Gain1 : Gain  Gain=-1
  Saturation Dynamic : simulink/Discontinuities/Saturation Dynamic  OutMin=[]  OutMax=[]  OutDataTypeStr=Inherit: Same as second input  OutDataType=fixdt(1, 16)  OutScaling=2^-10  DoSatur=off
  Sum : Sum  Inputs=|++
  Sum1 : Sum  Inputs=-+|
  Switch : Switch  Criteria=u2 > Threshold
  Unit Delay : UnitDelay  SampleTime=-1  HasFrameUpgradeWarning=on
  out : Outport  VectorParamsAs1DForOutWhenUnconnected=off
  wires:
  Switch/1 -> Unit Delay/1
  Sum/1 -> Switch/3
  Saturation Dynamic/1 -> Sum/1
  in/1 -> Sum1/2
  Sum1/1 -> Saturation Dynamic/2
  rst/1 -> Switch/2
  init/1 -> Switch/1
  Unit Delay/1 -> Sum/2, Sum1/1, out/1
  rate/1 -> Gain/1
  Gain/1 -> Saturation Dynamic/1, Gain1/1
  Gain1/1 -> Saturation Dynamic/3

== system Auto_microgrid_forecasting/MODEL STABILIZER/AllStringInverters/Stab_control/InvControl/CB_Meas2/Filter ==
  In1 : Inport
  Discrete 2nd-Order Filter : powerlib_extras/Discrete  Control Blocks/Discrete  2nd-Order Filter  FilterType=Lowpass  Fo=10  Zeta=0.707  Ts=Ts  Initialize=off  Vac_Init=[0.8 -25 60]  Vdc_Init=-0.4  PlotResponse=off  param1=[1 500 1]
      settings: SourceProductBaseCode=PS
  Discrete 2nd-Order Filter1 : powerlib_extras/Discrete  Control Blocks/Discrete  2nd-Order Filter  FilterType=Lowpass  Fo=10  Zeta=0.707  Ts=Ts  Initialize=off  Vac_Init=[0.8 -25 60]  Vdc_Init=-0.4  PlotResponse=off  param1=[1 500 1]
      settings: SourceProductBaseCode=PS
  Mux : Mux  Inputs=2
  Selector1 : Selector  InputPortWidth=3  IndexOptions=Index vector (dialog)  Indices=1  OutputSizes=1
  Selector2 : Selector  InputPortWidth=3  IndexOptions=Index vector (dialog)  Indices=2  OutputSizes=1
  Out1 : Outport  VectorParamsAs1DForOutWhenUnconnected=off
  wires:
  In1/1 -> Selector2/1, Selector1/1
  Selector2/1 -> Discrete 2nd-Order Filter1/1
  Selector1/1 -> Discrete 2nd-Order Filter/1
  Discrete 2nd-Order Filter/1 -> Mux/1
  Discrete 2nd-Order Filter1/1 -> Mux/2
  Mux/1 -> Out1/1  "vdq0_line_flt"

== system Auto_microgrid_forecasting/MODEL STABILIZER/AllStringInverters/Stab_control/InvControl/CB_Meas2/Filter1 ==
  In1 : Inport
  Discrete 2nd-Order Filter : powerlib_extras/Discrete  Control Blocks/Discrete  2nd-Order Filter  FilterType=Lowpass  Fo=10  Zeta=0.707  Ts=Ts  Initialize=off  Vac_Init=[0.8 -25 60]  Vdc_Init=-0.4  PlotResponse=off  param1=[1 500 1]
      settings: SourceProductBaseCode=PS
  Discrete 2nd-Order Filter1 : powerlib_extras/Discrete  Control Blocks/Discrete  2nd-Order Filter  FilterType=Lowpass  Fo=10  Zeta=0.707  Ts=Ts  Initialize=off  Vac_Init=[0.8 -25 60]  Vdc_Init=-0.4  PlotResponse=off  param1=[1 500 1]
      settings: SourceProductBaseCode=PS
  Mux : Mux  Inputs=2
  Selector1 : Selector  InputPortWidth=3  IndexOptions=Index vector (dialog)  Indices=1  OutputSizes=1
  Selector2 : Selector  InputPortWidth=3  IndexOptions=Index vector (dialog)  Indices=2  OutputSizes=1
  Out1 : Outport  VectorParamsAs1DForOutWhenUnconnected=off
  wires:
  In1/1 -> Selector2/1, Selector1/1
  Selector2/1 -> Discrete 2nd-Order Filter1/1
  Selector1/1 -> Discrete 2nd-Order Filter/1
  Discrete 2nd-Order Filter/1 -> Mux/1
  Discrete 2nd-Order Filter1/1 -> Mux/2
  Mux/1 -> Out1/1  "idq0_line_flt"

== system Auto_microgrid_forecasting/MODEL STABILIZER/AllStringInverters/Stab_control/InvControl/CB_Meas2/PQ_Calculator ==
  note: Copyright (c) 2016 Massachusetts Institute of Technology
      | Permission is hereby granted, free of charge, to any person obtaining a copy of this software and associated documentation files (the "Software"), to deal
      | in the Software without restriction, including without limitation the rights to use, copy, modify, merge, publish, distribute, sublicense, and/or sell copies of the
      | Software, and to permit persons to whom the Software is furnished to do so, subject to the following conditions:
      |
      | THE SOFTWARE IS PROVIDED "AS IS", WITHOUT WARRANTY OF ANY KIND, EXPRESS OR IMPLIED, INCLUDING BUT NOT LIMITED TO THE
      | WARRANTIES OF MERCHANTABILITY, FITNESS FOR A PARTICULAR PURPOSE AND NONINFRINGEMENT. IN NO EVENT SHALL THE AUTHORS
      | OR COPYRIGHT HOLDERS BE LIABLE FOR ANY CLAIM, DAMAGES OR OTHER LIABILITY, WHETHER IN AN ACTION OF CONTRACT, TORT OR
      | OTHERWISE, ARISING FROM, OUT OF OR IN CONNECTION WITH THE SOFTWARE OR THE USE OR OTHER DEALINGS IN THE SOFTWARE
  Vabc : Inport
  Iabc : Inport  Port=2
  3-phase Instantaneous Active & Reactive Power : powerlib_extras/Measurements/3-phase  Instantaneous  Active & Reactive Power
      settings: SourceProductBaseCode=PS
  Demux : Demux  Outputs=2
  Discrete Mean value2 : powerlib_extras/Discrete Measurements/Discrete  Mean value  Freq=60  Vinit=0  Ts=Ts
      settings: SourceProductBaseCode=PS
  Gain10 : Gain  Gain=2/3
  Scope : Scope  NumInputPorts=4
  P - kW : Outport  VectorParamsAs1DForOutWhenUnconnected=off
  Q - kVAR : Outport  Port=2  VectorParamsAs1DForOutWhenUnconnected=off
  wires:
  Demux/2 -> Q - kVAR/1  "kvar"
  Demux/1 -> P - kW/1  "kw"
  Iabc/1 -> 3-phase Instantaneous Active & Reactive Power/2, Scope/2
  Vabc/1 -> 3-phase Instantaneous Active & Reactive Power/1, Scope/1
  Discrete Mean value2/1 -> Gain10/1
  3-phase Instantaneous Active & Reactive Power/1 -> Discrete Mean value2/1, Scope/3
  Gain10/1 -> Demux/1, Scope/4

== system Auto_microgrid_forecasting/MODEL STABILIZER/AllStringInverters/Stab_control/InvControl/Droop/Droop ==
  dfvpq : Inport
  droop : Inport  Port=2
  Constant4 : Constant  Value=2
  Dead Zone : DeadZone  LowerValue=-1.1  UpperValue=1.1  SaturateOnIntegerOverflow=on
  Demux : Demux
  Demux1 : Demux
  Discrete 1st-Order Filter : powerlib_extras/Discrete  Control Blocks/Discrete 1st-Order Filter  FilterType=Lowpass  Tc=1e-3  Ts=Ts  Initialize=off  Vac_Init=[0.8 -25 60]  Vdc_Init=-0.4  PlotResponse=off  param1=[1 500 0.1]
      settings: SourceProductBaseCode=PS
  Discrete 1st-Order Filter1 : powerlib_extras/Discrete  Control Blocks/Discrete 1st-Order Filter  FilterType=Lowpass  Tc=1e-3  Ts=Ts  Initialize=off  Vac_Init=[0.8 -25 60]  Vdc_Init=-0.4  PlotResponse=off  param1=[1 500 0.1]
      settings: SourceProductBaseCode=PS
  Discrete 2nd-Order Filter : powerlib_extras/Discrete  Control Blocks/Discrete  2nd-Order Filter  FilterType=Lowpass  Fo=100  Zeta=0.707  Ts=Ts  Initialize=off  Vac_Init=[0.8 -25 60]  Vdc_Init=-0.4  PlotResponse=off  param1=[1 500 1]
      settings: SourceProductBaseCode=PS
  Discrete 2nd-Order Filter1 : powerlib_extras/Discrete  Control Blocks/Discrete  2nd-Order Filter  FilterType=Lowpass  Fo=100  Zeta=0.707  Ts=Ts  Initialize=off  Vac_Init=[0.8 -25 60]  Vdc_Init=-0.4  PlotResponse=off  param1=[1 500 1]
      settings: SourceProductBaseCode=PS
  Mux1 : Mux
  Product{,1..4} (5 alike) : Product
  Selector : Selector  InputPortWidth=4  IndexOptions=Index vector (dialog)  Indices=[3 4 1 2]  OutputSizes=1
  Sum : Sum  Inputs=|++
  dFvpq_out : Outport  VectorParamsAs1DForOutWhenUnconnected=off
  wires:
  droop/1 -> Demux1/1
  Demux1/2 -> Product3/2
  Demux1/3 -> Product/2
  Demux1/4 -> Product2/2
  Demux1/1 -> Product1/2
  Mux1/1 -> Selector/1
  Product2/1 -> Sum/1  "v"
  Product/1 -> Mux1/3  "F"
  Product3/1 -> Mux1/2  "q"
  Product1/1 -> Mux1/1  "p"
  Demux/4 -> Discrete 2nd-Order Filter1/1  "q"
  Discrete 1st-Order Filter1/1 -> Product3/1
  Selector/1 -> dFvpq_out/1
  dfvpq/1 -> Demux/1
  Demux/1 -> Discrete 1st-Order Filter/1  "f"
  Demux/2 -> Discrete 1st-Order Filter1/1  "v"
  Discrete 1st-Order Filter/1 -> Product1/1
  Demux/3 -> Discrete 2nd-Order Filter/1  "p"
  Discrete 2nd-Order Filter1/1 -> Product2/1, Dead Zone/1
  Discrete 2nd-Order Filter/1 -> Product/1
  Dead Zone/1 -> Product4/1
  Constant4/1 -> Product4/2
  Sum/1 -> Mux1/4
  Product4/1 -> Sum/2

== system Auto_microgrid_forecasting/MODEL STABILIZER/AllStringInverters/Stab_control/InvControl/Droop/ExtractCoefs ==
  In1 : Inport
  Bus Selector8 : BusSelector  OutputSignals=FP_droop,VQ_droop,FP_droop,VQ_droop
  Mux : Mux
  Out1 : Outport  VectorParamsAs1DForOutWhenUnconnected=off
  wires:
  In1/1 -> Bus Selector8/1
  Mux/1 -> Out1/1
  Bus Selector8/3 -> Mux/3  "<FP_droop>"
  Bus Selector8/2 -> Mux/2  "<VQ_droop>"
  Bus Selector8/4 -> Mux/4  "<VQ_droop>"
  Bus Selector8/1 -> Mux/1  "<FP_droop>"

== system Auto_microgrid_forecasting/MODEL STABILIZER/AllStringInverters/Stab_control/InvControl/PLL/DebounceAlternative ==
  In : Inport
  Rst : Inport  Port=2
  Bias : Bias  Bias=-0.5
  Constant1 : Constant  Value=2/Tdb_on
  Constant2 : Constant  Value=2/Tdb_off
  Data Type Conversion : DataTypeConversion
  Delay : Delay  DelayLength=1  InitialCondition=0
  Discrete-Time Integrator : DiscreteIntegrator  IntegratorMethod=Accumulation: Forward Euler  gainval=Tdb_sample  ExternalReset=level  InitialConditionSource=external  InitialCondition=-0.001  SampleTime=Tdb_sample  OutDataTypeStr=double  LimitOutput=on  UpperSaturationLimit=1.001  LowerSaturationLimit=-0.001  ICPrevOutput=DiscIntNeverNeededParam  ICPrevScaledInput=DiscIntNeverNeededParam
  Logical Operator : Logic  Operator=NXOR  AllPortsSameDT=off  OutDataTypeStr=boolean
  Logical Operator1 : Logic  Operator=OR  AllPortsSameDT=off  OutDataTypeStr=boolean
  Logical Operator2 : Logic  Operator=NOT  AllPortsSameDT=off  OutDataTypeStr=boolean
  Logical Operator3 : Logic  AllPortsSameDT=off  OutDataTypeStr=boolean
  Product : Product
  Relay : Relay  OnSwitchValue=1  OffSwitchValue=0
  Switch : Switch  Threshold=0.5
  Out : Outport  VectorParamsAs1DForOutWhenUnconnected=off
  IntOut : Outport  Port=2  VectorParamsAs1DForOutWhenUnconnected=off
  wires:
  Data Type Conversion/1 -> Discrete-Time Integrator/3
  Logical Operator2/1 -> Logical Operator3/1
  Logical Operator3/1 -> Data Type Conversion/1
  Rst/1 -> Logical Operator1/2, Logical Operator2/1
  Logical Operator1/1 -> Discrete-Time Integrator/2
  In/1 -> Bias/1, Logical Operator/1
  Switch/1 -> Product/2
  Logical Operator/1 -> Logical Operator1/1
  Delay/1 -> Logical Operator/2, Logical Operator3/2, Switch/2
  Constant2/1 -> Switch/3
  Constant1/1 -> Switch/1
  Bias/1 -> Product/1
  Discrete-Time Integrator/1 -> IntOut/1, Relay/1
  Relay/1 -> Delay/1, Out/1
  Product/1 -> Discrete-Time Integrator/1

== system Auto_microgrid_forecasting/MODEL STABILIZER/AllStringInverters/Stab_control/InvControl/PLL/PLL (3ph)1 ==
  abc : Inport  PortDimensions=3
  Discrete : Subsystem  DialogController=POWERSYS.PowerSysDialog  mask(Discrete PID Controller){Kp=ParK(1), Ki=ParK(2), Kd=ParK(3), TcD=TcD, Par_Limits=[Flim(2) Flim(1)]*2*pi, Init=2*pi*Par_Init(2), Ts=Ts}
      mask prompts: Kp "Proportional gain (Kp):"; Ki "Integral gain (Ki):"; Kd "Derivative gain (Kd):"; TcD "Time constant for derivative filter (s):"; Par_Limits "Output limits: [ Upper   Lower ]"; Init "Output initial value:"; Ts "Sample time:"
      mask help: This block implements a discrete PID controller.
      mask Display: disp('PID');
  Discrete 2nd-Order Filter : powerlib_extras/Discrete  Control Blocks/Discrete  2nd-Order Filter  FilterType=Lowpass  Fo=10  Zeta=0.707  Ts=Ts  Initialize=off  Vac_Init=[0.8 -25 60]  Vdc_Init=-0.4  PlotResponse=off  param1=[1 500 1]
      settings: SourceProductBaseCode=PS
  Gain10 : Gain  Gain=1/2/pi  SaturateOnIntegerOverflow=on  OutDataTypeStr=Inherit: Same as input  ParamDataTypeStr=Inherit: Same as input
  Mux3 : Mux  Inputs=2
  Scope : Scope  NumInputPorts=4
  Selector : Selector  InputPortWidth=3  IndexOptions=Index vector (dialog)  Indices=2  OutputSizes=1
  Trigonometric Function2 : Trigonometry
  Trigonometric Function3 : Trigonometry  Operator=cos
  Unit Delay : UnitDelay  SampleTime=Ts  HasFrameUpgradeWarning=on
  VCO : Subsystem
  abc_to_dq0 Transformation : powerlib_extras/Measurements/abc_to_dq0 Transformation
      settings: SourceProductBaseCode=PS
  Freq : Outport  VectorParamsAs1DForOutWhenUnconnected=off
  wt : Outport  Port=2  VectorParamsAs1DForOutWhenUnconnected=off
  dq0 : Outport  Port=3  VectorParamsAs1DForOutWhenUnconnected=off
  wires:
  VCO/1(theta) -> Scope/3, wt/1, Trigonometric Function3/1, Trigonometric Function2/1  "wt"
  Discrete/1(Out) -> Gain10/1, VCO/1(w), Scope/2  "W"
  Unit Delay/1 -> Freq/1
  Gain10/1 -> Discrete 2nd-Order Filter/1
  Selector/1 -> Discrete/1(Err), Scope/1  "Vq"
  Discrete 2nd-Order Filter/1 -> Unit Delay/1
  abc/1 -> abc_to_dq0 Transformation/1, Scope/4
  abc_to_dq0 Transformation/1 -> Selector/1, dq0/1
  Mux3/1 -> abc_to_dq0 Transformation/2  "ejwt"
  Trigonometric Function2/1 -> Mux3/1
  Trigonometric Function3/1 -> Mux3/2

== system Auto_microgrid_forecasting/MODEL STABILIZER/AllStringInverters/Stab_control/InvControl/PLL/VCO ==
  w : Inport
  rst : Inport  Port=2
  init : Inport  Port=3
  Compare To Constant : simulink/Logic and Bit Operations/Compare To Constant  relop=>=  const=pi  OutDataTypeStr=uint8
  Data Type Conversion : DataTypeConversion
  Gain : Gain  Gain=2*pi  OutDataTypeStr=double
  Gain2 : Gain  Gain=Ts  SaturateOnIntegerOverflow=on  OutDataTypeStr=Inherit: Same as input  ParamDataTypeStr=Inherit: Same as input
  Sum : Sum  Inputs=-++
  Switch : Switch  Threshold=0.5
  Unit Delay1 : UnitDelay  SampleTime=-1  HasFrameUpgradeWarning=on
  theta : Outport  VectorParamsAs1DForOutWhenUnconnected=off
  wires:
  w/1 -> Gain2/1
  Gain/1 -> Sum/1
  Compare To Constant/1 -> Data Type Conversion/1
  Unit Delay1/1 -> Sum/3, theta/1, Compare To Constant/1  "wt"
  Gain2/1 -> Sum/2
  Sum/1 -> Switch/3
  Switch/1 -> Unit Delay1/1
  rst/1 -> Switch/2
  init/1 -> Switch/1
  Data Type Conversion/1 -> Gain/1
